simulink model "SecRwRtStHdrstFwdBkwdTrgtPosSelc"  (R2018b)
settings: Solver=FixedStepDiscrete  StartTime=0.0  StopTime=10.0  FixedStep=0.01  RelTol=1e-3
undefined symbols (not defined in the file or in its folder): KeSMSw4SAcsMd23SecRwRtStHdrstFrwdBkwdPos_Val, KeSMSw4SAcsMd23SecRwRtStHdrstFrwdBkwdPosMax_Val, KeSMSw4SAcsMd23SecRwRtStHdrstFrwdBkwdPosMin_Val, KeSMSw4SAcsMd24SecRwRtStHdrstFrwdBkwdPos_Val, KeSMSw4SAcsMd24SecRwRtStHdrstFrwdBkwdPosMax_Val, KeSMSw4SAcsMd24SecRwRtStHdrstFrwdBkwdPosMin_Val, KeSMSw4SAcsMd25SecRwRtStHdrstFrwdBkwdPos_Val, KeSMSw4SAcsMd25SecRwRtStHdrstFrwdBkwdPosMax_Val, KeSMSw4SAcsMd25SecRwRtStHdrstFrwdBkwdPosMin_Val, KeSMSw4SAcsMd26SecRwRtStHdrstFrwdBkwdPos_Val, KeSMSw4SAcsMd26SecRwRtStHdrstFrwdBkwdPosMax_Val, KeSMSw4SAcsMd26SecRwRtStHdrstFrwdBkwdPosMin_Val, KeSMSw4sLyingMDSecRwRtStHdrstFrwdBkwdnwdPos_160_Val, KeSMSw4sLyingMDSecRwRtStHdrstFrwdBkwdnwdPos_165_Val, KeSMSw4sLyingMDSecRwRtStHdrstFrwdBkwdnwdPos_170_Val, KeSMSw4sLyingMDSecRwRtStHdrstFrwdBkwdnwdPos_175_Val, KeSMSw4sLyingMDSecRwRtStHdrstFrwdBkwdnwdPos_180_Val, KeSMSw4sLyingMDSecRwRtStHdrstFrwdBkwdnwdPos_Below160_Val, KeSMSw4sLyingMDSecRwRtStHdrstFrwdBkwdnwdPos_Over180_Val, KeSMSw4sLyingMDSecRwRtStHdrstFrwdBkwdnwdPosMax_160_Val, KeSMSw4sLyingMDSecRwRtStHdrstFrwdBkwdnwdPosMax_165_Val, KeSMSw4sLyingMDSecRwRtStHdrstFrwdBkwdnwdPosMax_170_Val, KeSMSw4sLyingMDSecRwRtStHdrstFrwdBkwdnwdPosMax_175_Val, KeSMSw4sLyingMDSecRwRtStHdrstFrwdBkwdnwdPosMax_180_Val, KeSMSw4sLyingMDSecRwRtStHdrstFrwdBkwdnwdPosMax_Below160_Val, KeSMSw4sLyingMDSecRwRtStHdrstFrwdBkwdnwdPosMax_Over180_Val, KeSMSw4sLyingMDSecRwRtStHdrstFrwdBkwdnwdPosMin_160_Val, KeSMSw4sLyingMDSecRwRtStHdrstFrwdBkwdnwdPosMin_165_Val, KeSMSw4sLyingMDSecRwRtStHdrstFrwdBkwdnwdPosMin_170_Val, KeSMSw4sLyingMDSecRwRtStHdrstFrwdBkwdnwdPosMin_175_Val, KeSMSw4sLyingMDSecRwRtStHdrstFrwdBkwdnwdPosMin_180_Val, KeSMSw4sLyingMDSecRwRtStHdrstFrwdBkwdnwdPosMin_Below160_Val, KeSMSw4sLyingMDSecRwRtStHdrstFrwdBkwdnwdPosMin_Over180_Val, KeSMSw4sRecoveryMDSecRwRtStHdrstFrwdBkwdPos_160_Val, KeSMSw4sRecoveryMDSecRwRtStHdrstFrwdBkwdPos_165_Val, KeSMSw4sRecoveryMDSecRwRtStHdrstFrwdBkwdPos_170_Val, KeSMSw4sRecoveryMDSecRwRtStHdrstFrwdBkwdPos_175_Val, KeSMSw4sRecoveryMDSecRwRtStHdrstFrwdBkwdPos_180_Val, KeSMSw4sRecoveryMDSecRwRtStHdrstFrwdBkwdPos_Below160_Val, KeSMSw4sRecoveryMDSecRwRtStHdrstFrwdBkwdPos_Over180_Val, KeSMSw4sRecoveryMDSecRwRtStHdrstFrwdBkwdPosMax_160_Val, KeSMSw4sRecoveryMDSecRwRtStHdrstFrwdBkwdPosMax_165_Val, KeSMSw4sRecoveryMDSecRwRtStHdrstFrwdBkwdPosMax_170_Val, KeSMSw4sRecoveryMDSecRwRtStHdrstFrwdBkwdPosMax_175_Val, KeSMSw4sRecoveryMDSecRwRtStHdrstFrwdBkwdPosMax_180_Val, KeSMSw4sRecoveryMDSecRwRtStHdrstFrwdBkwdPosMax_Below160_Val, KeSMSw4sRecoveryMDSecRwRtStHdrstFrwdBkwdPosMax_Over180_Val, KeSMSw4sRecoveryMDSecRwRtStHdrstFrwdBkwdPosMin_160_Val, KeSMSw4sRecoveryMDSecRwRtStHdrstFrwdBkwdPosMin_165_Val, KeSMSw4sRecoveryMDSecRwRtStHdrstFrwdBkwdPosMin_170_Val, KeSMSw4sRecoveryMDSecRwRtStHdrstFrwdBkwdPosMin_175_Val, KeSMSw4sRecoveryMDSecRwRtStHdrstFrwdBkwdPosMin_180_Val, KeSMSw4sRecoveryMDSecRwRtStHdrstFrwdBkwdPosMin_Below160_Val, KeSMSw4sRecoveryMDSecRwRtStHdrstFrwdBkwdPosMin_Over180_Val, KeSMSw4sVIPMDSecRwRtStHdrstFrwdBkwdPos_160_Val, KeSMSw4sVIPMDSecRwRtStHdrstFrwdBkwdPos_165_Val, KeSMSw4sVIPMDSecRwRtStHdrstFrwdBkwdPos_170_Val, KeSMSw4sVIPMDSecRwRtStHdrstFrwdBkwdPos_175_Val, KeSMSw4sVIPMDSecRwRtStHdrstFrwdBkwdPos_180_Val, KeSMSw4sVIPMDSecRwRtStHdrstFrwdBkwdPos_Below160_Val ... (+15)
libraries: TrgtPosSelcLib x4
settings Model: ModifiedHistory=2023.8.1 V2.0.0 CR401790 增加模式21-26  Creator=sn2xws  LastModifiedBy=sn2xws
settings DataIOCC: SaveFormat=StructureWithTime
settings OptimizationCC: DefaultParameterBehavior=Inlined  EnhancedBackFolding=on  PassReuseOutputArgsAs=Individual arguments  ZeroExternalMemoryAtStartup=off  ZeroInternalMemoryAtStartup=off  OptimizeBlockOrder=speed  DifferentSizesBufferReuse=on  OptimizationCustomize=off
settings DebuggingCC: ParameterTunabilityLossMsg=error
settings HardwareCC: ProdLongLongMode=on
settings ModelReferenceCC: ModelReferenceNumInstancesAllowed=Single
settings SFSimCC: MATLABDynamicMemAlloc=off
settings RTWCC: SystemTargetFile=autosar.tlc  GenCodeOnly=on  TemplateMakefile=ert_default_tmf  Description=AUTOSAR  GenerateReport=on  BuildConfiguration=Debug  IncludeHyperlinkInReport=on  LaunchReport=on  GenerateTraceInfo=on  GenerateTraceReport=on  GenerateTraceReportSl=on  GenerateTraceReportSf=on  GenerateTraceReportEml=on
settings CodeAppCC: ForceParamTrailComments=on  IgnoreCustomStorageClasses=off  OperatorAnnotations=on  SimulinkDataObjDesc=on  SFDataObjDesc=on  InsertBlockDesc=on
settings STFCustomTargetCC: TargetLangStandard=C99 (ISO)  MultiwordLength=256  ParMdlRefBuildCompliant=on  CompOptLevelCompliant=on  IncludeMdlTerminateFcn=off  CombineOutputUpdateFcns=on  SuppressErrorStatus=on  ERTCustomFileBanners=on  SupportNonFinite=off  SupportComplex=off  SupportContinuousTime=off  SupportNonInlinedSFcns=off  RemoveResetFunc=on  MATLABClassNameForMDSCustomization=Simulink.SoftwareTarget.ERTCustomization  AutosarCompliant=on  UseToolchainInfoCompliant=on  LookupTableObjectStructAxisOrder=2,1,3,4,...  LUTObjectStructOrderEvenSpacing=Size,Table,Breakpoints  SystemTargetFile=autosar.tlc
settings ERTTargetCC: TargetLangStandard=C99 (ISO)  ConcurrentExecutionCompliant=off  IncludeMdlTerminateFcn=off  SuppressErrorStatus=on  SupportNonFinite=off  SupportComplex=off  ModelStepFunctionPrototypeControlCompliant=off  CPPClassGenCompliant=off  AutosarCompliant=on  LookupTableObjectStructAxisOrder=2,1,3,4,...  LUTObjectStructOrderEvenSpacing=Size,Table,Breakpoints  InlinedParameterPlacement=NonHierarchical  ERTCustomFileTemplate=example_file_process.tlc  ERTFilePackagingFormat=Compact

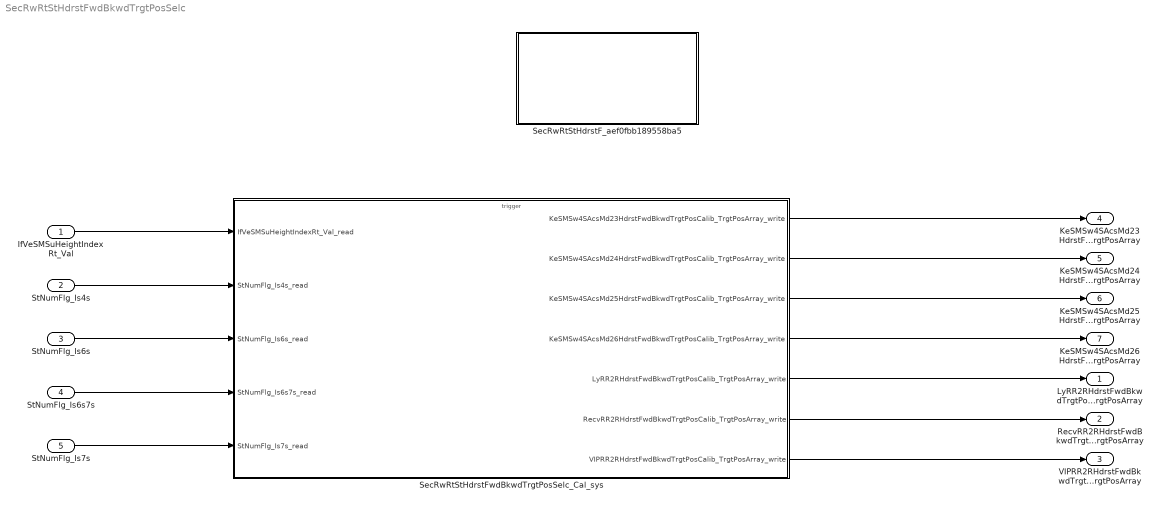
== system SecRwRtStHdrstFwdBkwdTrgtPosSelc ==
  IfVeSMSuHeightIndexRt_Val : Inport  Description=|  OutDataTypeStr=uint8  PortDimensions=1
      | 0：under 160
      | 1：160
      | 2：165
      | 3：170
      | 4：175
      | 5：180
      | 6：over 180
  StNumFlg_Is4s : Inport  Port=2  OutDataTypeStr=boolean  PortDimensions=1
  StNumFlg_Is6s : Inport  Port=3  OutDataTypeStr=boolean  PortDimensions=1
  StNumFlg_Is6s7s : Inport  Port=4  OutDataTypeStr=boolean  PortDimensions=1
  StNumFlg_Is7s : Inport  Port=5  OutDataTypeStr=boolean  PortDimensions=1
  SecRwRtStHdrstF_aef0fbb189558ba5 : Subsystem
  SecRwRtStHdrstFwdBkwdTrgtPosSelc_Cal_sys : Subsystem
  LyRR2RHdrstFwdBkwdTrgtPosCalib_TrgtPosArray : Outport  Description=|  OutDataTypeStr=uint16  PortDimensions=3
      | 0:Pos
      | 1:Max
      | 2:Min
  RecvRR2RHdrstFwdBkwdTrgtPosCalib_TrgtPosArray : Outport  Description=|  Port=2  OutDataTypeStr=uint16  PortDimensions=3
      | 0:Pos
      | 1:Max
      | 2:Min
  VIPRR2RHdrstFwdBkwdTrgtPosCalib_TrgtPosArray : Outport  Description=|  Port=3  OutDataTypeStr=uint16  PortDimensions=3
      | 0:Pos
      | 1:Max
      | 2:Min
  KeSMSw4SAcsMd23HdrstFwdBkwdTrgtPosCalib_TrgtPosArray : Outport  Description=|  Port=4  OutDataTypeStr=uint16  PortDimensions=3
      | 0:Pos
      | 1:Max
      | 2:Min
  KeSMSw4SAcsMd24HdrstFwdBkwdTrgtPosCalib_TrgtPosArray : Outport  Description=|  Port=5  OutDataTypeStr=uint16  PortDimensions=3
      | 0:Pos
      | 1:Max
      | 2:Min
  KeSMSw4SAcsMd25HdrstFwdBkwdTrgtPosCalib_TrgtPosArray : Outport  Description=|  Port=6  OutDataTypeStr=uint16  PortDimensions=3
      | 0:Pos
      | 1:Max
      | 2:Min
  KeSMSw4SAcsMd26HdrstFwdBkwdTrgtPosCalib_TrgtPosArray : Outport  Description=|  Port=7  OutDataTypeStr=uint16  PortDimensions=3
      | 0:Pos
      | 1:Max
      | 2:Min
  wires:
  IfVeSMSuHeightIndexRt_Val/1 -> SecRwRtStHdrstFwdBkwdTrgtPosSelc_Cal_sys/1(IfVeSMSuHeightIndexRt_Val_read)
  StNumFlg_Is4s/1 -> SecRwRtStHdrstFwdBkwdTrgtPosSelc_Cal_sys/2(StNumFlg_Is4s_read)
  StNumFlg_Is6s/1 -> SecRwRtStHdrstFwdBkwdTrgtPosSelc_Cal_sys/3(StNumFlg_Is6s_read)
  StNumFlg_Is6s7s/1 -> SecRwRtStHdrstFwdBkwdTrgtPosSelc_Cal_sys/4(StNumFlg_Is6s7s_read)
  StNumFlg_Is7s/1 -> SecRwRtStHdrstFwdBkwdTrgtPosSelc_Cal_sys/5(StNumFlg_Is7s_read)
  SecRwRtStHdrstFwdBkwdTrgtPosSelc_Cal_sys/5(LyRR2RHdrstFwdBkwdTrgtPosCalib_TrgtPosArray_write) -> LyRR2RHdrstFwdBkwdTrgtPosCalib_TrgtPosArray/1
  SecRwRtStHdrstFwdBkwdTrgtPosSelc_Cal_sys/6(RecvRR2RHdrstFwdBkwdTrgtPosCalib_TrgtPosArray_write) -> RecvRR2RHdrstFwdBkwdTrgtPosCalib_TrgtPosArray/1
  SecRwRtStHdrstFwdBkwdTrgtPosSelc_Cal_sys/7(VIPRR2RHdrstFwdBkwdTrgtPosCalib_TrgtPosArray_write) -> VIPRR2RHdrstFwdBkwdTrgtPosCalib_TrgtPosArray/1
  SecRwRtStHdrstFwdBkwdTrgtPosSelc_Cal_sys/1(KeSMSw4SAcsMd23HdrstFwdBkwdTrgtPosCalib_TrgtPosArray_write) -> KeSMSw4SAcsMd23HdrstFwdBkwdTrgtPosCalib_TrgtPosArray/1
  SecRwRtStHdrstFwdBkwdTrgtPosSelc_Cal_sys/2(KeSMSw4SAcsMd24HdrstFwdBkwdTrgtPosCalib_TrgtPosArray_write) -> KeSMSw4SAcsMd24HdrstFwdBkwdTrgtPosCalib_TrgtPosArray/1
  SecRwRtStHdrstFwdBkwdTrgtPosSelc_Cal_sys/3(KeSMSw4SAcsMd25HdrstFwdBkwdTrgtPosCalib_TrgtPosArray_write) -> KeSMSw4SAcsMd25HdrstFwdBkwdTrgtPosCalib_TrgtPosArray/1
  SecRwRtStHdrstFwdBkwdTrgtPosSelc_Cal_sys/4(KeSMSw4SAcsMd26HdrstFwdBkwdTrgtPosCalib_TrgtPosArray_write) -> KeSMSw4SAcsMd26HdrstFwdBkwdTrgtPosCalib_TrgtPosArray/1

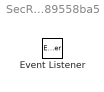
== system SecRwRtStHdrstFwdBkwdTrgtPosSelc/SecRwRtStHdrstF_aef0fbb189558ba5 ==
  Event Listener : EventListener  EventName=reset

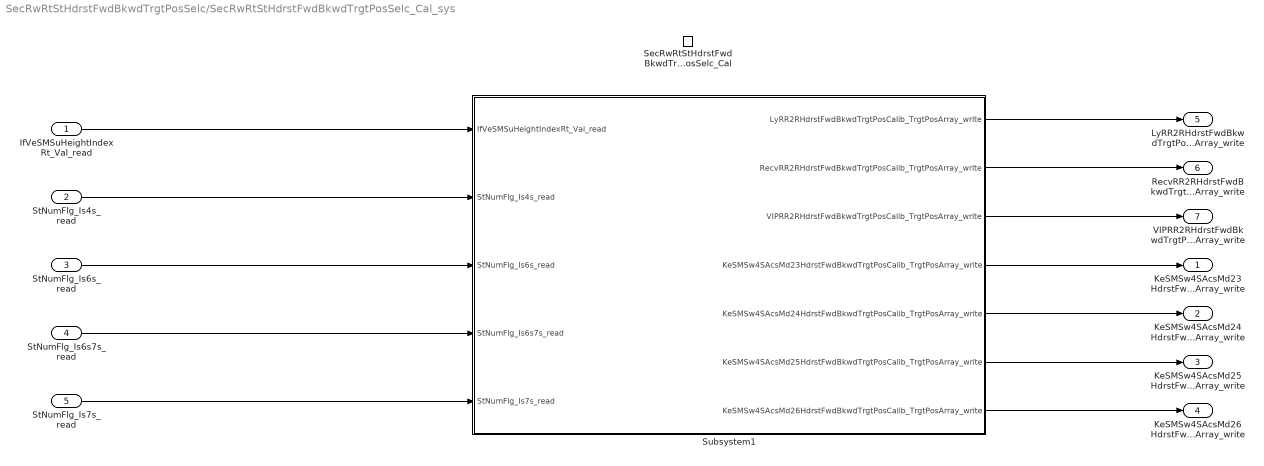
== system SecRwRtStHdrstFwdBkwdTrgtPosSelc/SecRwRtStHdrstFwdBkwdTrgtPosSelc_Cal_sys ==
  IfVeSMSuHeightIndexRt_Val_read : Inport
  StNumFlg_Is4s_read : Inport  Port=2
  StNumFlg_Is6s_read : Inport  Port=3
  StNumFlg_Is6s7s_read : Inport  Port=4
  StNumFlg_Is7s_read : Inport  Port=5
  SecRwRtStHdrstFwdBkwdTrgtPosSelc_Cal : TriggerPort  TriggerType=function-call  IsSimulinkFunction=on  FunctionName=SecRwRtStHdrstFwdBkwdTrgtPosSelc_Cal  VariantControl=(inherit)
  Subsystem1 : Subsystem
  KeSMSw4SAcsMd23HdrstFwdBkwdTrgtPosCalib_TrgtPosArray_write : Outport
      settings: EnsureOutportIsVirtual=on
  KeSMSw4SAcsMd24HdrstFwdBkwdTrgtPosCalib_TrgtPosArray_write : Outport  Port=2
      settings: EnsureOutportIsVirtual=on
  KeSMSw4SAcsMd25HdrstFwdBkwdTrgtPosCalib_TrgtPosArray_write : Outport  Port=3
      settings: EnsureOutportIsVirtual=on
  KeSMSw4SAcsMd26HdrstFwdBkwdTrgtPosCalib_TrgtPosArray_write : Outport  Port=4
      settings: EnsureOutportIsVirtual=on
  LyRR2RHdrstFwdBkwdTrgtPosCalib_TrgtPosArray_write : Outport  Port=5
      settings: EnsureOutportIsVirtual=on
  RecvRR2RHdrstFwdBkwdTrgtPosCalib_TrgtPosArray_write : Outport  Port=6
      settings: EnsureOutportIsVirtual=on
  VIPRR2RHdrstFwdBkwdTrgtPosCalib_TrgtPosArray_write : Outport  Port=7
      settings: EnsureOutportIsVirtual=on
  wires:
  Subsystem1/1(LyRR2RHdrstFwdBkwdTrgtPosCalib_TrgtPosArray_write) -> LyRR2RHdrstFwdBkwdTrgtPosCalib_TrgtPosArray_write/1
  Subsystem1/2(RecvRR2RHdrstFwdBkwdTrgtPosCalib_TrgtPosArray_write) -> RecvRR2RHdrstFwdBkwdTrgtPosCalib_TrgtPosArray_write/1
  Subsystem1/3(VIPRR2RHdrstFwdBkwdTrgtPosCalib_TrgtPosArray_write) -> VIPRR2RHdrstFwdBkwdTrgtPosCalib_TrgtPosArray_write/1
  Subsystem1/4(KeSMSw4SAcsMd23HdrstFwdBkwdTrgtPosCalib_TrgtPosArray_write) -> KeSMSw4SAcsMd23HdrstFwdBkwdTrgtPosCalib_TrgtPosArray_write/1
  Subsystem1/5(KeSMSw4SAcsMd24HdrstFwdBkwdTrgtPosCalib_TrgtPosArray_write) -> KeSMSw4SAcsMd24HdrstFwdBkwdTrgtPosCalib_TrgtPosArray_write/1
  Subsystem1/6(KeSMSw4SAcsMd25HdrstFwdBkwdTrgtPosCalib_TrgtPosArray_write) -> KeSMSw4SAcsMd25HdrstFwdBkwdTrgtPosCalib_TrgtPosArray_write/1
  Subsystem1/7(KeSMSw4SAcsMd26HdrstFwdBkwdTrgtPosCalib_TrgtPosArray_write) -> KeSMSw4SAcsMd26HdrstFwdBkwdTrgtPosCalib_TrgtPosArray_write/1
  StNumFlg_Is4s_read/1 -> Subsystem1/2(StNumFlg_Is4s_read)
  StNumFlg_Is6s_read/1 -> Subsystem1/3(StNumFlg_Is6s_read)
  IfVeSMSuHeightIndexRt_Val_read/1 -> Subsystem1/1(IfVeSMSuHeightIndexRt_Val_read)
  StNumFlg_Is6s7s_read/1 -> Subsystem1/4(StNumFlg_Is6s7s_read)
  StNumFlg_Is7s_read/1 -> Subsystem1/5(StNumFlg_Is7s_read)

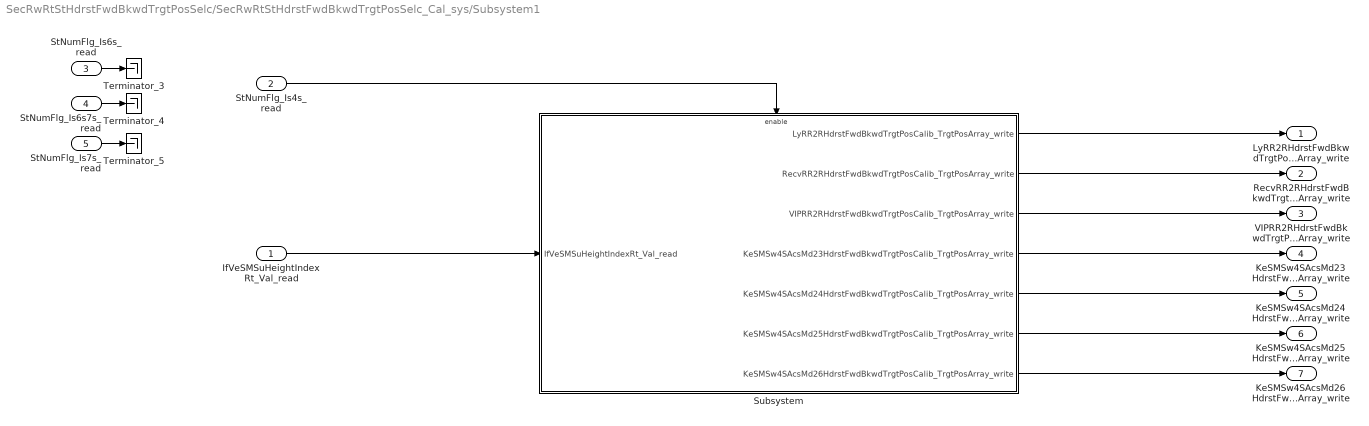
== system SecRwRtStHdrstFwdBkwdTrgtPosSelc/SecRwRtStHdrstFwdBkwdTrgtPosSelc_Cal_sys/Subsystem1 ==
  IfVeSMSuHeightIndexRt_Val_read : Inport
  StNumFlg_Is4s_read : Inport  Port=2
  StNumFlg_Is6s_read : Inport  Port=3
  StNumFlg_Is6s7s_read : Inport  Port=4
  StNumFlg_Is7s_read : Inport  Port=5
  Subsystem : Subsystem
  Terminator_3 : Terminator
  Terminator_4 : Terminator
  Terminator_5 : Terminator
  LyRR2RHdrstFwdBkwdTrgtPosCalib_TrgtPosArray_write : Outport
      settings: EnsureOutportIsVirtual=on
  RecvRR2RHdrstFwdBkwdTrgtPosCalib_TrgtPosArray_write : Outport  Port=2
      settings: EnsureOutportIsVirtual=on
  VIPRR2RHdrstFwdBkwdTrgtPosCalib_TrgtPosArray_write : Outport  Port=3
      settings: EnsureOutportIsVirtual=on
  KeSMSw4SAcsMd23HdrstFwdBkwdTrgtPosCalib_TrgtPosArray_write : Outport  Port=4
      settings: EnsureOutportIsVirtual=on
  KeSMSw4SAcsMd24HdrstFwdBkwdTrgtPosCalib_TrgtPosArray_write : Outport  Port=5
      settings: EnsureOutportIsVirtual=on
  KeSMSw4SAcsMd25HdrstFwdBkwdTrgtPosCalib_TrgtPosArray_write : Outport  Port=6
      settings: EnsureOutportIsVirtual=on
  KeSMSw4SAcsMd26HdrstFwdBkwdTrgtPosCalib_TrgtPosArray_write : Outport  Port=7
      settings: EnsureOutportIsVirtual=on
  wires:
  StNumFlg_Is4s_read/1 -> Subsystem/Enable
  Subsystem/2(RecvRR2RHdrstFwdBkwdTrgtPosCalib_TrgtPosArray_write) -> RecvRR2RHdrstFwdBkwdTrgtPosCalib_TrgtPosArray_write/1
  StNumFlg_Is6s7s_read/1 -> Terminator_4/1
  IfVeSMSuHeightIndexRt_Val_read/1 -> Subsystem/1(IfVeSMSuHeightIndexRt_Val_read)
  StNumFlg_Is6s_read/1 -> Terminator_3/1
  Subsystem/1(LyRR2RHdrstFwdBkwdTrgtPosCalib_TrgtPosArray_write) -> LyRR2RHdrstFwdBkwdTrgtPosCalib_TrgtPosArray_write/1
  Subsystem/3(VIPRR2RHdrstFwdBkwdTrgtPosCalib_TrgtPosArray_write) -> VIPRR2RHdrstFwdBkwdTrgtPosCalib_TrgtPosArray_write/1
  StNumFlg_Is7s_read/1 -> Terminator_5/1
  Subsystem/7(KeSMSw4SAcsMd26HdrstFwdBkwdTrgtPosCalib_TrgtPosArray_write) -> KeSMSw4SAcsMd26HdrstFwdBkwdTrgtPosCalib_TrgtPosArray_write/1
  Subsystem/4(KeSMSw4SAcsMd23HdrstFwdBkwdTrgtPosCalib_TrgtPosArray_write) -> KeSMSw4SAcsMd23HdrstFwdBkwdTrgtPosCalib_TrgtPosArray_write/1
  Subsystem/5(KeSMSw4SAcsMd24HdrstFwdBkwdTrgtPosCalib_TrgtPosArray_write) -> KeSMSw4SAcsMd24HdrstFwdBkwdTrgtPosCalib_TrgtPosArray_write/1
  Subsystem/6(KeSMSw4SAcsMd25HdrstFwdBkwdTrgtPosCalib_TrgtPosArray_write) -> KeSMSw4SAcsMd25HdrstFwdBkwdTrgtPosCalib_TrgtPosArray_write/1

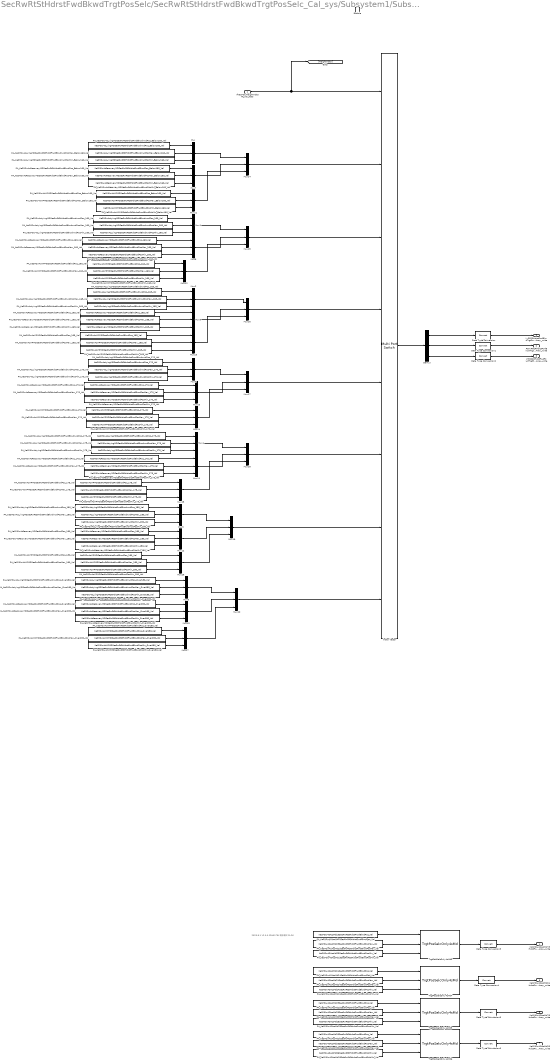
== system SecRwRtStHdrstFwdBkwdTrgtPosSelc/SecRwRtStHdrstFwdBkwdTrgtPosSelc_Cal_sys/Subsystem1/Subsystem ==
  note: 2023.8.1 V2.0.0 CR401790 增加模式21-26
  IfVeSMSuHeightIndexRt_Val_read : Inport
  Enable : EnablePort
  Data Type Conversion{,1..6} (7 alike) : DataTypeConversion
  Demux : Demux  Outputs=3
  Index Vector : MultiPortSwitch  DataPortOrder=Zero-based contiguous  Inputs=7  DiagnosticForDefault=None  zeroidx=on
  Mux{,1..27} (28 alike) : Mux  Inputs=3
  PA_KeSMSw4SAcsMd23SecRwRtStHdrstFrwdBkwdPosMax_Val : Constant  Value=KeSMSw4SAcsMd23SecRwRtStHdrstFrwdBkwdPosMax_Val
  PA_KeSMSw4SAcsMd23SecRwRtStHdrstFrwdBkwdPosMin_Val : Constant  Value=KeSMSw4SAcsMd23SecRwRtStHdrstFrwdBkwdPosMin_Val
  PA_KeSMSw4SAcsMd23SecRwRtStHdrstFrwdBkwdPos_Val : Constant  Value=KeSMSw4SAcsMd23SecRwRtStHdrstFrwdBkwdPos_Val
  PA_KeSMSw4SAcsMd24SecRwRtStHdrstFrwdBkwdPosMax_Val : Constant  Value=KeSMSw4SAcsMd24SecRwRtStHdrstFrwdBkwdPosMax_Val
  PA_KeSMSw4SAcsMd24SecRwRtStHdrstFrwdBkwdPosMin_Val : Constant  Value=KeSMSw4SAcsMd24SecRwRtStHdrstFrwdBkwdPosMin_Val
  PA_KeSMSw4SAcsMd24SecRwRtStHdrstFrwdBkwdPos_Val : Constant  Value=KeSMSw4SAcsMd24SecRwRtStHdrstFrwdBkwdPos_Val
  PA_KeSMSw4SAcsMd25SecRwRtStHdrstFrwdBkwdPosMax_Val : Constant  Value=KeSMSw4SAcsMd25SecRwRtStHdrstFrwdBkwdPosMax_Val
  PA_KeSMSw4SAcsMd25SecRwRtStHdrstFrwdBkwdPosMin_Val : Constant  Value=KeSMSw4SAcsMd25SecRwRtStHdrstFrwdBkwdPosMin_Val
  PA_KeSMSw4SAcsMd25SecRwRtStHdrstFrwdBkwdPos_Val : Constant  Value=KeSMSw4SAcsMd25SecRwRtStHdrstFrwdBkwdPos_Val
  PA_KeSMSw4SAcsMd26SecRwRtStHdrstFrwdBkwdPosMax_Val : Constant  Value=KeSMSw4SAcsMd26SecRwRtStHdrstFrwdBkwdPosMax_Val
  PA_KeSMSw4SAcsMd26SecRwRtStHdrstFrwdBkwdPosMin_Val : Constant  Value=KeSMSw4SAcsMd26SecRwRtStHdrstFrwdBkwdPosMin_Val
  PA_KeSMSw4SAcsMd26SecRwRtStHdrstFrwdBkwdPos_Val : Constant  Value=KeSMSw4SAcsMd26SecRwRtStHdrstFrwdBkwdPos_Val
  PA_KeSMSw4sLyingMDSecRwRtStHdrstFrwdBkwdnwdPosMax_160_Val : Constant  Value=KeSMSw4sLyingMDSecRwRtStHdrstFrwdBkwdnwdPosMax_160_Val
  PA_KeSMSw4sLyingMDSecRwRtStHdrstFrwdBkwdnwdPosMax_165_Val : Constant  Value=KeSMSw4sLyingMDSecRwRtStHdrstFrwdBkwdnwdPosMax_165_Val
  PA_KeSMSw4sLyingMDSecRwRtStHdrstFrwdBkwdnwdPosMax_170_Val : Constant  Value=KeSMSw4sLyingMDSecRwRtStHdrstFrwdBkwdnwdPosMax_170_Val
  PA_KeSMSw4sLyingMDSecRwRtStHdrstFrwdBkwdnwdPosMax_175_Val : Constant  Value=KeSMSw4sLyingMDSecRwRtStHdrstFrwdBkwdnwdPosMax_175_Val
  PA_KeSMSw4sLyingMDSecRwRtStHdrstFrwdBkwdnwdPosMax_180_Val : Constant  Value=KeSMSw4sLyingMDSecRwRtStHdrstFrwdBkwdnwdPosMax_180_Val
  PA_KeSMSw4sLyingMDSecRwRtStHdrstFrwdBkwdnwdPosMax_Below160_Val : Constant  Value=KeSMSw4sLyingMDSecRwRtStHdrstFrwdBkwdnwdPosMax_Below160_Val
  PA_KeSMSw4sLyingMDSecRwRtStHdrstFrwdBkwdnwdPosMax_Over180_Val : Constant  Value=KeSMSw4sLyingMDSecRwRtStHdrstFrwdBkwdnwdPosMax_Over180_Val
  PA_KeSMSw4sLyingMDSecRwRtStHdrstFrwdBkwdnwdPosMin_160_Val : Constant  Value=KeSMSw4sLyingMDSecRwRtStHdrstFrwdBkwdnwdPosMin_160_Val
  PA_KeSMSw4sLyingMDSecRwRtStHdrstFrwdBkwdnwdPosMin_165_Val : Constant  Value=KeSMSw4sLyingMDSecRwRtStHdrstFrwdBkwdnwdPosMin_165_Val
  PA_KeSMSw4sLyingMDSecRwRtStHdrstFrwdBkwdnwdPosMin_170_Val : Constant  Value=KeSMSw4sLyingMDSecRwRtStHdrstFrwdBkwdnwdPosMin_170_Val
  PA_KeSMSw4sLyingMDSecRwRtStHdrstFrwdBkwdnwdPosMin_175_Val : Constant  Value=KeSMSw4sLyingMDSecRwRtStHdrstFrwdBkwdnwdPosMin_175_Val
  PA_KeSMSw4sLyingMDSecRwRtStHdrstFrwdBkwdnwdPosMin_180_Val : Constant  Value=KeSMSw4sLyingMDSecRwRtStHdrstFrwdBkwdnwdPosMin_180_Val
  PA_KeSMSw4sLyingMDSecRwRtStHdrstFrwdBkwdnwdPosMin_Below160_Val : Constant  Value=KeSMSw4sLyingMDSecRwRtStHdrstFrwdBkwdnwdPosMin_Below160_Val
  PA_KeSMSw4sLyingMDSecRwRtStHdrstFrwdBkwdnwdPosMin_Over180_Val : Constant  Value=KeSMSw4sLyingMDSecRwRtStHdrstFrwdBkwdnwdPosMin_Over180_Val
  PA_KeSMSw4sLyingMDSecRwRtStHdrstFrwdBkwdnwdPos_160_Val : Constant  Value=KeSMSw4sLyingMDSecRwRtStHdrstFrwdBkwdnwdPos_160_Val
  PA_KeSMSw4sLyingMDSecRwRtStHdrstFrwdBkwdnwdPos_165_Val : Constant  Value=KeSMSw4sLyingMDSecRwRtStHdrstFrwdBkwdnwdPos_165_Val
  PA_KeSMSw4sLyingMDSecRwRtStHdrstFrwdBkwdnwdPos_170_Val : Constant  Value=KeSMSw4sLyingMDSecRwRtStHdrstFrwdBkwdnwdPos_170_Val
  PA_KeSMSw4sLyingMDSecRwRtStHdrstFrwdBkwdnwdPos_175_Val : Constant  Value=KeSMSw4sLyingMDSecRwRtStHdrstFrwdBkwdnwdPos_175_Val
  PA_KeSMSw4sLyingMDSecRwRtStHdrstFrwdBkwdnwdPos_180_Val : Constant  Value=KeSMSw4sLyingMDSecRwRtStHdrstFrwdBkwdnwdPos_180_Val
  PA_KeSMSw4sLyingMDSecRwRtStHdrstFrwdBkwdnwdPos_Below160_Val : Constant  Value=KeSMSw4sLyingMDSecRwRtStHdrstFrwdBkwdnwdPos_Below160_Val
  PA_KeSMSw4sLyingMDSecRwRtStHdrstFrwdBkwdnwdPos_Over180_Val : Constant  Value=KeSMSw4sLyingMDSecRwRtStHdrstFrwdBkwdnwdPos_Over180_Val
  PA_KeSMSw4sRecoveryMDSecRwRtStHdrstFrwdBkwdPosMax_160_Val : Constant  Value=KeSMSw4sRecoveryMDSecRwRtStHdrstFrwdBkwdPosMax_160_Val
  PA_KeSMSw4sRecoveryMDSecRwRtStHdrstFrwdBkwdPosMax_165_Val : Constant  Value=KeSMSw4sRecoveryMDSecRwRtStHdrstFrwdBkwdPosMax_165_Val
  PA_KeSMSw4sRecoveryMDSecRwRtStHdrstFrwdBkwdPosMax_170_Val : Constant  Value=KeSMSw4sRecoveryMDSecRwRtStHdrstFrwdBkwdPosMax_170_Val
  PA_KeSMSw4sRecoveryMDSecRwRtStHdrstFrwdBkwdPosMax_175_Val : Constant  Value=KeSMSw4sRecoveryMDSecRwRtStHdrstFrwdBkwdPosMax_175_Val
  PA_KeSMSw4sRecoveryMDSecRwRtStHdrstFrwdBkwdPosMax_180_Val : Constant  Value=KeSMSw4sRecoveryMDSecRwRtStHdrstFrwdBkwdPosMax_180_Val
  PA_KeSMSw4sRecoveryMDSecRwRtStHdrstFrwdBkwdPosMax_Below160_Val : Constant  Value=KeSMSw4sRecoveryMDSecRwRtStHdrstFrwdBkwdPosMax_Below160_Val
  PA_KeSMSw4sRecoveryMDSecRwRtStHdrstFrwdBkwdPosMax_Over180_Val : Constant  Value=KeSMSw4sRecoveryMDSecRwRtStHdrstFrwdBkwdPosMax_Over180_Val
  PA_KeSMSw4sRecoveryMDSecRwRtStHdrstFrwdBkwdPosMin_160_Val : Constant  Value=KeSMSw4sRecoveryMDSecRwRtStHdrstFrwdBkwdPosMin_160_Val
  PA_KeSMSw4sRecoveryMDSecRwRtStHdrstFrwdBkwdPosMin_165_Val : Constant  Value=KeSMSw4sRecoveryMDSecRwRtStHdrstFrwdBkwdPosMin_165_Val
  PA_KeSMSw4sRecoveryMDSecRwRtStHdrstFrwdBkwdPosMin_170_Val : Constant  Value=KeSMSw4sRecoveryMDSecRwRtStHdrstFrwdBkwdPosMin_170_Val
  PA_KeSMSw4sRecoveryMDSecRwRtStHdrstFrwdBkwdPosMin_175_Val : Constant  Value=KeSMSw4sRecoveryMDSecRwRtStHdrstFrwdBkwdPosMin_175_Val
  PA_KeSMSw4sRecoveryMDSecRwRtStHdrstFrwdBkwdPosMin_180_Val : Constant  Value=KeSMSw4sRecoveryMDSecRwRtStHdrstFrwdBkwdPosMin_180_Val
  PA_KeSMSw4sRecoveryMDSecRwRtStHdrstFrwdBkwdPosMin_Below160_Val : Constant  Value=KeSMSw4sRecoveryMDSecRwRtStHdrstFrwdBkwdPosMin_Below160_Val
  PA_KeSMSw4sRecoveryMDSecRwRtStHdrstFrwdBkwdPosMin_Over180_Val : Constant  Value=KeSMSw4sRecoveryMDSecRwRtStHdrstFrwdBkwdPosMin_Over180_Val
  PA_KeSMSw4sRecoveryMDSecRwRtStHdrstFrwdBkwdPos_160_Val : Constant  Value=KeSMSw4sRecoveryMDSecRwRtStHdrstFrwdBkwdPos_160_Val
  PA_KeSMSw4sRecoveryMDSecRwRtStHdrstFrwdBkwdPos_165_Val : Constant  Value=KeSMSw4sRecoveryMDSecRwRtStHdrstFrwdBkwdPos_165_Val
  PA_KeSMSw4sRecoveryMDSecRwRtStHdrstFrwdBkwdPos_170_Val : Constant  Value=KeSMSw4sRecoveryMDSecRwRtStHdrstFrwdBkwdPos_170_Val
  PA_KeSMSw4sRecoveryMDSecRwRtStHdrstFrwdBkwdPos_175_Val : Constant  Value=KeSMSw4sRecoveryMDSecRwRtStHdrstFrwdBkwdPos_175_Val
  PA_KeSMSw4sRecoveryMDSecRwRtStHdrstFrwdBkwdPos_180_Val : Constant  Value=KeSMSw4sRecoveryMDSecRwRtStHdrstFrwdBkwdPos_180_Val
  PA_KeSMSw4sRecoveryMDSecRwRtStHdrstFrwdBkwdPos_Below160_Val : Constant  Value=KeSMSw4sRecoveryMDSecRwRtStHdrstFrwdBkwdPos_Below160_Val
  PA_KeSMSw4sRecoveryMDSecRwRtStHdrstFrwdBkwdPos_Over180_Val : Constant  Value=KeSMSw4sRecoveryMDSecRwRtStHdrstFrwdBkwdPos_Over180_Val
  PA_KeSMSw4sVIPMDSecRwRtStHdrstFrwdBkwdPosMax_160_Val : Constant  Value=KeSMSw4sVIPMDSecRwRtStHdrstFrwdBkwdPosMax_160_Val
  PA_KeSMSw4sVIPMDSecRwRtStHdrstFrwdBkwdPosMax_165_Val : Constant  Value=KeSMSw4sVIPMDSecRwRtStHdrstFrwdBkwdPosMax_165_Val
  PA_KeSMSw4sVIPMDSecRwRtStHdrstFrwdBkwdPosMax_170_Val : Constant  Value=KeSMSw4sVIPMDSecRwRtStHdrstFrwdBkwdPosMax_170_Val
  PA_KeSMSw4sVIPMDSecRwRtStHdrstFrwdBkwdPosMax_175_Val : Constant  Value=KeSMSw4sVIPMDSecRwRtStHdrstFrwdBkwdPosMax_175_Val
  PA_KeSMSw4sVIPMDSecRwRtStHdrstFrwdBkwdPosMax_180_Val : Constant  Value=KeSMSw4sVIPMDSecRwRtStHdrstFrwdBkwdPosMax_180_Val
  PA_KeSMSw4sVIPMDSecRwRtStHdrstFrwdBkwdPosMax_Below160_Val : Constant  Value=KeSMSw4sVIPMDSecRwRtStHdrstFrwdBkwdPosMax_Below160_Val
  PA_KeSMSw4sVIPMDSecRwRtStHdrstFrwdBkwdPosMax_Over180_Val : Constant  Value=KeSMSw4sVIPMDSecRwRtStHdrstFrwdBkwdPosMax_Over180_Val
  PA_KeSMSw4sVIPMDSecRwRtStHdrstFrwdBkwdPosMin_160_Val : Constant  Value=KeSMSw4sVIPMDSecRwRtStHdrstFrwdBkwdPosMin_160_Val
  PA_KeSMSw4sVIPMDSecRwRtStHdrstFrwdBkwdPosMin_165_Val : Constant  Value=KeSMSw4sVIPMDSecRwRtStHdrstFrwdBkwdPosMin_165_Val
  PA_KeSMSw4sVIPMDSecRwRtStHdrstFrwdBkwdPosMin_170_Val : Constant  Value=KeSMSw4sVIPMDSecRwRtStHdrstFrwdBkwdPosMin_170_Val
  PA_KeSMSw4sVIPMDSecRwRtStHdrstFrwdBkwdPosMin_175_Val : Constant  Value=KeSMSw4sVIPMDSecRwRtStHdrstFrwdBkwdPosMin_175_Val
  PA_KeSMSw4sVIPMDSecRwRtStHdrstFrwdBkwdPosMin_180_Val : Constant  Value=KeSMSw4sVIPMDSecRwRtStHdrstFrwdBkwdPosMin_180_Val
  PA_KeSMSw4sVIPMDSecRwRtStHdrstFrwdBkwdPosMin_Below160_Val : Constant  Value=KeSMSw4sVIPMDSecRwRtStHdrstFrwdBkwdPosMin_Below160_Val
  PA_KeSMSw4sVIPMDSecRwRtStHdrstFrwdBkwdPosMin_Over180_Val : Constant  Value=KeSMSw4sVIPMDSecRwRtStHdrstFrwdBkwdPosMin_Over180_Val
  PA_KeSMSw4sVIPMDSecRwRtStHdrstFrwdBkwdPos_160_Val : Constant  Value=KeSMSw4sVIPMDSecRwRtStHdrstFrwdBkwdPos_160_Val
  PA_KeSMSw4sVIPMDSecRwRtStHdrstFrwdBkwdPos_165_Val : Constant  Value=KeSMSw4sVIPMDSecRwRtStHdrstFrwdBkwdPos_165_Val
  PA_KeSMSw4sVIPMDSecRwRtStHdrstFrwdBkwdPos_170_Val : Constant  Value=KeSMSw4sVIPMDSecRwRtStHdrstFrwdBkwdPos_170_Val
  PA_KeSMSw4sVIPMDSecRwRtStHdrstFrwdBkwdPos_175_Val : Constant  Value=KeSMSw4sVIPMDSecRwRtStHdrstFrwdBkwdPos_175_Val
  PA_KeSMSw4sVIPMDSecRwRtStHdrstFrwdBkwdPos_180_Val : Constant  Value=KeSMSw4sVIPMDSecRwRtStHdrstFrwdBkwdPos_180_Val
  PA_KeSMSw4sVIPMDSecRwRtStHdrstFrwdBkwdPos_Below160_Val : Constant  Value=KeSMSw4sVIPMDSecRwRtStHdrstFrwdBkwdPos_Below160_Val
  PA_KeSMSw4sVIPMDSecRwRtStHdrstFrwdBkwdPos_Over180_Val : Constant  Value=KeSMSw4sVIPMDSecRwRtStHdrstFrwdBkwdPos_Over180_Val
  TrgtPosSelcOnly4sMd{3..6} (4 alike) : TrgtPosSelcLib/TrgtPosSelcOnly4sMd  SystemSampleTime=-1
  LyRR2RHdrstFwdBkwdTrgtPosCalib_TrgtPosArray_write : Outport
  RecvRR2RHdrstFwdBkwdTrgtPosCalib_TrgtPosArray_write : Outport  Port=2
  VIPRR2RHdrstFwdBkwdTrgtPosCalib_TrgtPosArray_write : Outport  Port=3
  KeSMSw4SAcsMd23HdrstFwdBkwdTrgtPosCalib_TrgtPosArray_write : Outport  Port=4
  KeSMSw4SAcsMd24HdrstFwdBkwdTrgtPosCalib_TrgtPosArray_write : Outport  Port=5
  KeSMSw4SAcsMd25HdrstFwdBkwdTrgtPosCalib_TrgtPosArray_write : Outport  Port=6
  KeSMSw4SAcsMd26HdrstFwdBkwdTrgtPosCalib_TrgtPosArray_write : Outport  Port=7
  wires:
  IfVeSMSuHeightIndexRt_Val_read/1 -> [HeightIndex], Index Vector/1
  Demux/3 -> Data Type Conversion2/1
  Data Type Conversion/1 -> LyRR2RHdrstFwdBkwdTrgtPosCalib_TrgtPosArray_write/1
  Data Type Conversion1/1 -> RecvRR2RHdrstFwdBkwdTrgtPosCalib_TrgtPosArray_write/1
  Data Type Conversion2/1 -> VIPRR2RHdrstFwdBkwdTrgtPosCalib_TrgtPosArray_write/1
  TrgtPosSelcOnly4sMd3/1 -> Data Type Conversion3/1
  TrgtPosSelcOnly4sMd4/1 -> Data Type Conversion4/1
  TrgtPosSelcOnly4sMd5/1 -> Data Type Conversion5/1
  TrgtPosSelcOnly4sMd6/1 -> Data Type Conversion6/1
  PA_KeSMSw4SAcsMd23SecRwRtStHdrstFrwdBkwdPosMax_Val/1 -> TrgtPosSelcOnly4sMd3/2
  PA_KeSMSw4SAcsMd23SecRwRtStHdrstFrwdBkwdPosMin_Val/1 -> TrgtPosSelcOnly4sMd3/3
  PA_KeSMSw4SAcsMd23SecRwRtStHdrstFrwdBkwdPos_Val/1 -> TrgtPosSelcOnly4sMd3/1
  PA_KeSMSw4SAcsMd24SecRwRtStHdrstFrwdBkwdPosMax_Val/1 -> TrgtPosSelcOnly4sMd4/2
  PA_KeSMSw4SAcsMd24SecRwRtStHdrstFrwdBkwdPosMin_Val/1 -> TrgtPosSelcOnly4sMd4/3
  PA_KeSMSw4SAcsMd24SecRwRtStHdrstFrwdBkwdPos_Val/1 -> TrgtPosSelcOnly4sMd4/1
  PA_KeSMSw4SAcsMd25SecRwRtStHdrstFrwdBkwdPosMax_Val/1 -> TrgtPosSelcOnly4sMd5/2
  PA_KeSMSw4SAcsMd25SecRwRtStHdrstFrwdBkwdPosMin_Val/1 -> TrgtPosSelcOnly4sMd5/3
  PA_KeSMSw4SAcsMd25SecRwRtStHdrstFrwdBkwdPos_Val/1 -> TrgtPosSelcOnly4sMd5/1
  PA_KeSMSw4SAcsMd26SecRwRtStHdrstFrwdBkwdPosMax_Val/1 -> TrgtPosSelcOnly4sMd6/2
  PA_KeSMSw4SAcsMd26SecRwRtStHdrstFrwdBkwdPosMin_Val/1 -> TrgtPosSelcOnly4sMd6/3
  PA_KeSMSw4SAcsMd26SecRwRtStHdrstFrwdBkwdPos_Val/1 -> TrgtPosSelcOnly4sMd6/1
  Data Type Conversion3/1 -> KeSMSw4SAcsMd23HdrstFwdBkwdTrgtPosCalib_TrgtPosArray_write/1
  Data Type Conversion4/1 -> KeSMSw4SAcsMd24HdrstFwdBkwdTrgtPosCalib_TrgtPosArray_write/1
  Data Type Conversion5/1 -> KeSMSw4SAcsMd25HdrstFwdBkwdTrgtPosCalib_TrgtPosArray_write/1
  Data Type Conversion6/1 -> KeSMSw4SAcsMd26HdrstFwdBkwdTrgtPosCalib_TrgtPosArray_write/1
  PA_KeSMSw4sLyingMDSecRwRtStHdrstFrwdBkwdnwdPosMin_Below160_Val/1 -> Mux/3
  PA_KeSMSw4sLyingMDSecRwRtStHdrstFrwdBkwdnwdPosMax_Below160_Val/1 -> Mux/2
  PA_KeSMSw4sLyingMDSecRwRtStHdrstFrwdBkwdnwdPos_Below160_Val/1 -> Mux/1
  PA_KeSMSw4sLyingMDSecRwRtStHdrstFrwdBkwdnwdPosMax_160_Val/1 -> Mux1/2
  PA_KeSMSw4sLyingMDSecRwRtStHdrstFrwdBkwdnwdPosMin_160_Val/1 -> Mux1/3
  PA_KeSMSw4sLyingMDSecRwRtStHdrstFrwdBkwdnwdPos_160_Val/1 -> Mux1/1
  PA_KeSMSw4sLyingMDSecRwRtStHdrstFrwdBkwdnwdPosMax_165_Val/1 -> Mux2/2
  PA_KeSMSw4sLyingMDSecRwRtStHdrstFrwdBkwdnwdPosMin_165_Val/1 -> Mux2/3
  PA_KeSMSw4sLyingMDSecRwRtStHdrstFrwdBkwdnwdPos_165_Val/1 -> Mux2/1
  PA_KeSMSw4sLyingMDSecRwRtStHdrstFrwdBkwdnwdPosMax_170_Val/1 -> Mux3/2
  PA_KeSMSw4sLyingMDSecRwRtStHdrstFrwdBkwdnwdPosMin_170_Val/1 -> Mux3/3
  PA_KeSMSw4sLyingMDSecRwRtStHdrstFrwdBkwdnwdPos_170_Val/1 -> Mux3/1
  PA_KeSMSw4sLyingMDSecRwRtStHdrstFrwdBkwdnwdPosMax_175_Val/1 -> Mux4/2
  PA_KeSMSw4sLyingMDSecRwRtStHdrstFrwdBkwdnwdPosMin_175_Val/1 -> Mux4/3
  PA_KeSMSw4sLyingMDSecRwRtStHdrstFrwdBkwdnwdPos_175_Val/1 -> Mux4/1
  PA_KeSMSw4sLyingMDSecRwRtStHdrstFrwdBkwdnwdPosMax_180_Val/1 -> Mux5/2
  PA_KeSMSw4sLyingMDSecRwRtStHdrstFrwdBkwdnwdPosMin_180_Val/1 -> Mux5/3
  PA_KeSMSw4sLyingMDSecRwRtStHdrstFrwdBkwdnwdPos_180_Val/1 -> Mux5/1
  PA_KeSMSw4sLyingMDSecRwRtStHdrstFrwdBkwdnwdPosMax_Over180_Val/1 -> Mux6/2
  PA_KeSMSw4sLyingMDSecRwRtStHdrstFrwdBkwdnwdPosMin_Over180_Val/1 -> Mux6/3
  PA_KeSMSw4sLyingMDSecRwRtStHdrstFrwdBkwdnwdPos_Over180_Val/1 -> Mux6/1
  PA_KeSMSw4sRecoveryMDSecRwRtStHdrstFrwdBkwdPos_Below160_Val/1 -> Mux7/1
  PA_KeSMSw4sRecoveryMDSecRwRtStHdrstFrwdBkwdPosMax_Below160_Val/1 -> Mux7/2
  PA_KeSMSw4sRecoveryMDSecRwRtStHdrstFrwdBkwdPosMin_Below160_Val/1 -> Mux7/3
  PA_KeSMSw4sRecoveryMDSecRwRtStHdrstFrwdBkwdPosMax_160_Val/1 -> Mux8/2
  PA_KeSMSw4sRecoveryMDSecRwRtStHdrstFrwdBkwdPosMin_160_Val/1 -> Mux8/3
  PA_KeSMSw4sRecoveryMDSecRwRtStHdrstFrwdBkwdPos_160_Val/1 -> Mux8/1
  PA_KeSMSw4sRecoveryMDSecRwRtStHdrstFrwdBkwdPosMax_165_Val/1 -> Mux9/2
  PA_KeSMSw4sRecoveryMDSecRwRtStHdrstFrwdBkwdPosMin_165_Val/1 -> Mux9/3
  PA_KeSMSw4sRecoveryMDSecRwRtStHdrstFrwdBkwdPos_165_Val/1 -> Mux9/1
  PA_KeSMSw4sRecoveryMDSecRwRtStHdrstFrwdBkwdPosMax_170_Val/1 -> Mux10/2
  PA_KeSMSw4sRecoveryMDSecRwRtStHdrstFrwdBkwdPos_170_Val/1 -> Mux10/1
  PA_KeSMSw4sRecoveryMDSecRwRtStHdrstFrwdBkwdPosMin_170_Val/1 -> Mux10/3
  PA_KeSMSw4sRecoveryMDSecRwRtStHdrstFrwdBkwdPosMax_175_Val/1 -> Mux11/2
  PA_KeSMSw4sRecoveryMDSecRwRtStHdrstFrwdBkwdPosMin_175_Val/1 -> Mux11/3
  PA_KeSMSw4sRecoveryMDSecRwRtStHdrstFrwdBkwdPos_175_Val/1 -> Mux11/1
  PA_KeSMSw4sRecoveryMDSecRwRtStHdrstFrwdBkwdPosMax_180_Val/1 -> Mux12/2
  PA_KeSMSw4sRecoveryMDSecRwRtStHdrstFrwdBkwdPosMin_180_Val/1 -> Mux12/3
  PA_KeSMSw4sRecoveryMDSecRwRtStHdrstFrwdBkwdPos_180_Val/1 -> Mux12/1
  PA_KeSMSw4sRecoveryMDSecRwRtStHdrstFrwdBkwdPosMax_Over180_Val/1 -> Mux13/2
  PA_KeSMSw4sRecoveryMDSecRwRtStHdrstFrwdBkwdPosMin_Over180_Val/1 -> Mux13/3
  PA_KeSMSw4sRecoveryMDSecRwRtStHdrstFrwdBkwdPos_Over180_Val/1 -> Mux13/1
  Mux/1 -> Mux14/1
  Mux7/1 -> Mux14/2
  Mux14/1 -> Index Vector/2
  Mux15/1 -> Index Vector/3
  Mux16/1 -> Index Vector/4
  Mux17/1 -> Index Vector/5
  Mux18/1 -> Index Vector/6
  Mux19/1 -> Index Vector/7
  Mux20/1 -> Index Vector/8
  Mux6/1 -> Mux20/1
  Mux13/1 -> Mux20/2
  Mux5/1 -> Mux19/1
  Mux12/1 -> Mux19/2
  Mux4/1 -> Mux18/1
  Mux11/1 -> Mux18/2
  Mux3/1 -> Mux17/1
  Mux10/1 -> Mux17/2
  Mux2/1 -> Mux16/1
  Mux9/1 -> Mux16/2
  Mux1/1 -> Mux15/1
  Mux8/1 -> Mux15/2
  Index Vector/1 -> Demux/1
  Demux/1 -> Data Type Conversion/1
  Demux/2 -> Data Type Conversion1/1
  PA_KeSMSw4sVIPMDSecRwRtStHdrstFrwdBkwdPosMax_Below160_Val/1 -> Mux21/2
  PA_KeSMSw4sVIPMDSecRwRtStHdrstFrwdBkwdPosMin_Below160_Val/1 -> Mux21/3
  PA_KeSMSw4sVIPMDSecRwRtStHdrstFrwdBkwdPos_Below160_Val/1 -> Mux21/1
  PA_KeSMSw4sVIPMDSecRwRtStHdrstFrwdBkwdPosMax_160_Val/1 -> Mux22/2
  PA_KeSMSw4sVIPMDSecRwRtStHdrstFrwdBkwdPosMin_160_Val/1 -> Mux22/3
  PA_KeSMSw4sVIPMDSecRwRtStHdrstFrwdBkwdPos_160_Val/1 -> Mux22/1
  PA_KeSMSw4sVIPMDSecRwRtStHdrstFrwdBkwdPosMax_165_Val/1 -> Mux23/2
  PA_KeSMSw4sVIPMDSecRwRtStHdrstFrwdBkwdPosMin_165_Val/1 -> Mux23/3
  PA_KeSMSw4sVIPMDSecRwRtStHdrstFrwdBkwdPos_165_Val/1 -> Mux23/1
  PA_KeSMSw4sVIPMDSecRwRtStHdrstFrwdBkwdPosMax_170_Val/1 -> Mux24/2
  PA_KeSMSw4sVIPMDSecRwRtStHdrstFrwdBkwdPosMin_170_Val/1 -> Mux24/3
  PA_KeSMSw4sVIPMDSecRwRtStHdrstFrwdBkwdPos_170_Val/1 -> Mux24/1
  PA_KeSMSw4sVIPMDSecRwRtStHdrstFrwdBkwdPosMax_175_Val/1 -> Mux25/2
  PA_KeSMSw4sVIPMDSecRwRtStHdrstFrwdBkwdPosMin_175_Val/1 -> Mux25/3
  PA_KeSMSw4sVIPMDSecRwRtStHdrstFrwdBkwdPos_175_Val/1 -> Mux25/1
  PA_KeSMSw4sVIPMDSecRwRtStHdrstFrwdBkwdPosMax_180_Val/1 -> Mux26/2
  PA_KeSMSw4sVIPMDSecRwRtStHdrstFrwdBkwdPosMin_180_Val/1 -> Mux26/3
  PA_KeSMSw4sVIPMDSecRwRtStHdrstFrwdBkwdPos_180_Val/1 -> Mux26/1
  PA_KeSMSw4sVIPMDSecRwRtStHdrstFrwdBkwdPosMax_Over180_Val/1 -> Mux27/2
  PA_KeSMSw4sVIPMDSecRwRtStHdrstFrwdBkwdPosMin_Over180_Val/1 -> Mux27/3
  PA_KeSMSw4sVIPMDSecRwRtStHdrstFrwdBkwdPos_Over180_Val/1 -> Mux27/1
  Mux27/1 -> Mux20/3
  Mux26/1 -> Mux19/3
  Mux25/1 -> Mux18/3
  Mux24/1 -> Mux17/3
  Mux23/1 -> Mux16/3
  Mux22/1 -> Mux15/3
  Mux21/1 -> Mux14/3
